simulink model "elevator"  (R2020a)
settings: Solver=VariableStepAuto  StartTime=0.0  StopTime=inf  RelTol=1e-3
PreLoadFcn:
  | slplc.api.loadDataTypes;
undefined symbols (not defined in the file): BOOL, DINT, INT, slplc
libraries: simulink x1
(part 1 of 38)
settings Model: Creator=Ishmael  LastModifiedBy=ieatg

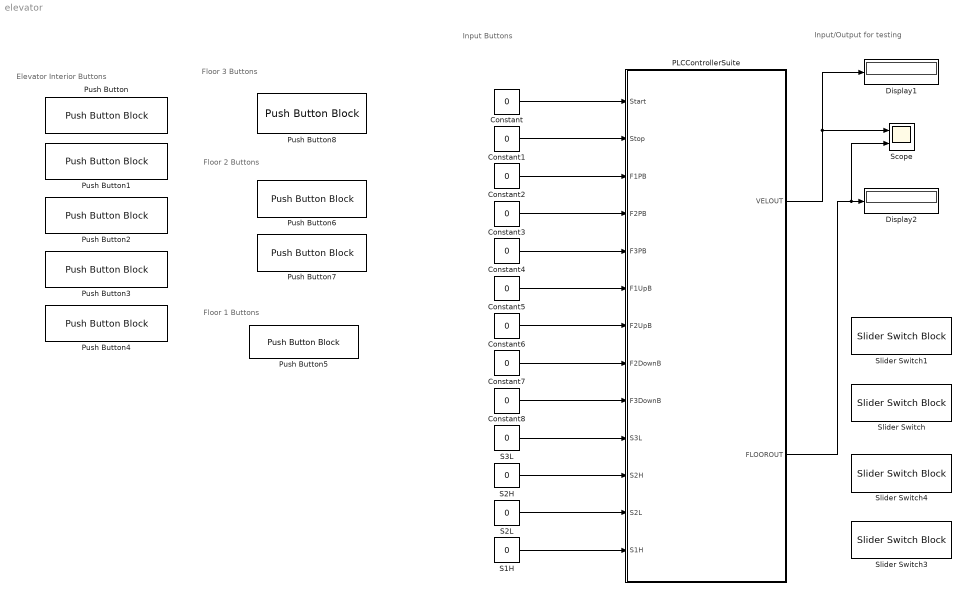
== system elevator ==
  note: Input/Output for testing
  note: Input Buttons
  note: Floor 2 Buttons
  note: Floor 3 Buttons
  note: Floor 1 Buttons
  note: Elevator Interior Buttons
  Constant{,1..8} (9 alike) : Constant  Value=0  OutDataTypeStr=BOOL
  Display1 : Display
  Display2 : Display
  PLCControllerSuite : Subsystem  TreatAsAtomicUnit=on  mask{PLCBlockType=PLCController, PLCPOUType=PLC Controller}
      mask init:
      | slplc.callbacks.initController(gcb);
      settings: OpenFcn=slplc.callbacks.openPOUBlock(gcb);
      mask Help: web([docroot '/plccoder/ref/plccontrollersuite' '.html']);
      mask DialogControl PLCBlockTitle Prompt: PLC Controller Block
  Push Button : PushButtonBlock  ButtonText=StartButton
  Push Button1 : PushButtonBlock  ButtonText=Stop
  Push Button2 : PushButtonBlock  ButtonText=Floor 1 PB
  Push Button3 : PushButtonBlock  ButtonText=Floor 2 PB
  Push Button4 : PushButtonBlock  ButtonText=Floor 3 PB
  Push Button5 : PushButtonBlock  ButtonText=Up Button Floor 1
  Push Button6 : PushButtonBlock  ButtonText=Up Button Floor 2
  Push Button7 : PushButtonBlock  ButtonText=Down Button Floor 2
  Push Button8 : PushButtonBlock  ButtonText=Down Button Floor 3
  S1H : Constant  Value=0  OutDataTypeStr=BOOL
  S2H : Constant  Value=0  OutDataTypeStr=BOOL
  S2L : Constant  Value=0  OutDataTypeStr=BOOL
  S3L : Constant  Value=0  OutDataTypeStr=BOOL
  Scope : Scope  NumInputPorts=2
  Slider Switch{,1,3..4} (4 alike) : SliderSwitchBlock
      settings: Values={{'Off', 'On'}, [0 1]}
  wires:
  Constant/1 -> PLCControllerSuite/1(Start)
  Constant1/1 -> PLCControllerSuite/2(Stop)
  Constant2/1 -> PLCControllerSuite/3(F1PB)
  Constant3/1 -> PLCControllerSuite/4(F2PB)
  Constant4/1 -> PLCControllerSuite/5(F3PB)
  Constant5/1 -> PLCControllerSuite/6(F1UpB)
  Constant6/1 -> PLCControllerSuite/7(F2UpB)
  Constant8/1 -> PLCControllerSuite/9(F3DownB)
  Constant7/1 -> PLCControllerSuite/8(F2DownB)
  PLCControllerSuite/1(VELOUT) -> Display1/1, Scope/1
  S3L/1 -> PLCControllerSuite/10(S3L)
  S2H/1 -> PLCControllerSuite/11(S2H)
  S2L/1 -> PLCControllerSuite/12(S2L)
  S1H/1 -> PLCControllerSuite/13(S1H)
  PLCControllerSuite/2(FLOOROUT) -> Scope/2, Display2/1

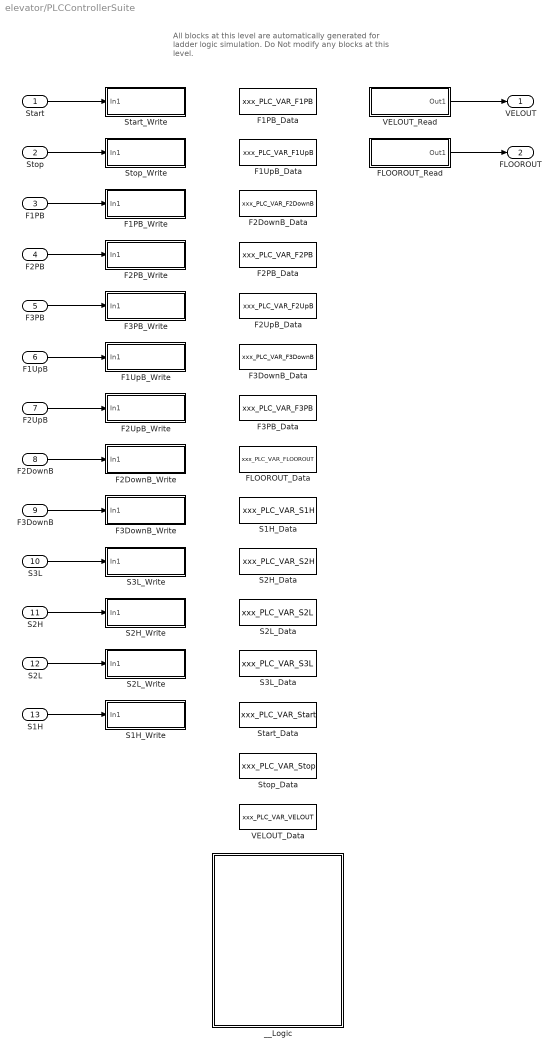
== system elevator/PLCControllerSuite ==
  note: All blocks at this level are automatically generated for ladder logic simulation.
      | Do Not modify any blocks at this level.
  Start : Inport  OutDataTypeStr=BOOL
  Stop : Inport  Port=2  OutDataTypeStr=BOOL
  F1PB : Inport  Port=3  OutDataTypeStr=BOOL
  F2PB : Inport  Port=4  OutDataTypeStr=BOOL
  F3PB : Inport  Port=5  OutDataTypeStr=BOOL
  F1UpB : Inport  Port=6  OutDataTypeStr=BOOL
  F2UpB : Inport  Port=7  OutDataTypeStr=BOOL
  F2DownB : Inport  Port=8  OutDataTypeStr=BOOL
  F3DownB : Inport  Port=9  OutDataTypeStr=BOOL
  S3L : Inport  Port=10  OutDataTypeStr=BOOL
  S2H : Inport  Port=11  OutDataTypeStr=BOOL
  S2L : Inport  Port=12  OutDataTypeStr=BOOL
  S1H : Inport  Port=13  OutDataTypeStr=BOOL
  F1PB_Data : DataStoreMemory  Tag=POUVariable  Priority=10  DataStoreName=xxx_PLC_VAR_F1PB  ShowAdditionalParam=off  OutDataTypeStr=BOOL  Dimensions=1
  F1PB_Write : Subsystem  Priority=11  DisableCoverage=on  TreatAsAtomicUnit=on  mask{PLCOperandTag=F1PB, PLCOperandExpression=xxx_PLC_VAR_F1PB, PLCBlockType=VarWrite, PLCPOUType=VarWrite}
      mask prompts: PLCOperandTag "Operand Tag:"
      mask init:
      | slplc.callbacks.initInstruction(gcb);
      mask Help: web([docroot '/plccoder/ref/varwrite' '.html']);
      mask DialogControl PLCBlockTitle Prompt: Variable Write
      mask Display: disp(get_param(gcb, 'PLCOperandTag'));
  F1UpB_Data : DataStoreMemory  Tag=POUVariable  Priority=10  DataStoreName=xxx_PLC_VAR_F1UpB  ShowAdditionalParam=off  OutDataTypeStr=BOOL  Dimensions=1
  F1UpB_Write : Subsystem  Priority=11  DisableCoverage=on  TreatAsAtomicUnit=on  mask{PLCOperandTag=F1UpB, PLCOperandExpression=xxx_PLC_VAR_F1UpB, PLCBlockType=VarWrite, PLCPOUType=VarWrite}
      mask prompts: PLCOperandTag "Operand Tag:"
      mask init:
      | slplc.callbacks.initInstruction(gcb);
      mask Help: web([docroot '/plccoder/ref/varwrite' '.html']);
      mask DialogControl PLCBlockTitle Prompt: Variable Write
      mask Display: disp(get_param(gcb, 'PLCOperandTag'));
  F2DownB_Data : DataStoreMemory  Tag=POUVariable  Priority=10  DataStoreName=xxx_PLC_VAR_F2DownB  ShowAdditionalParam=off  OutDataTypeStr=BOOL  Dimensions=1
  F2DownB_Write : Subsystem  Priority=11  DisableCoverage=on  TreatAsAtomicUnit=on  mask{PLCOperandTag=F2DownB, PLCOperandExpression=xxx_PLC_VAR_F2DownB, PLCBlockType=VarWrite, PLCPOUType=VarWrite}
      mask prompts: PLCOperandTag "Operand Tag:"
      mask init:
      | slplc.callbacks.initInstruction(gcb);
      mask Help: web([docroot '/plccoder/ref/varwrite' '.html']);
      mask DialogControl PLCBlockTitle Prompt: Variable Write
      mask Display: disp(get_param(gcb, 'PLCOperandTag'));
  F2PB_Data : DataStoreMemory  Tag=POUVariable  Priority=10  DataStoreName=xxx_PLC_VAR_F2PB  ShowAdditionalParam=off  OutDataTypeStr=BOOL  Dimensions=1
  F2PB_Write : Subsystem  Priority=11  DisableCoverage=on  TreatAsAtomicUnit=on  mask{PLCOperandTag=F2PB, PLCOperandExpression=xxx_PLC_VAR_F2PB, PLCBlockType=VarWrite, PLCPOUType=VarWrite}
      mask prompts: PLCOperandTag "Operand Tag:"
      mask init:
      | slplc.callbacks.initInstruction(gcb);
      mask Help: web([docroot '/plccoder/ref/varwrite' '.html']);
      mask DialogControl PLCBlockTitle Prompt: Variable Write
      mask Display: disp(get_param(gcb, 'PLCOperandTag'));
  F2UpB_Data : DataStoreMemory  Tag=POUVariable  Priority=10  DataStoreName=xxx_PLC_VAR_F2UpB  ShowAdditionalParam=off  OutDataTypeStr=BOOL  Dimensions=1
  F2UpB_Write : Subsystem  Priority=11  DisableCoverage=on  TreatAsAtomicUnit=on  mask{PLCOperandTag=F2UpB, PLCOperandExpression=xxx_PLC_VAR_F2UpB, PLCBlockType=VarWrite, PLCPOUType=VarWrite}
      mask prompts: PLCOperandTag "Operand Tag:"
      mask init:
      | slplc.callbacks.initInstruction(gcb);
      mask Help: web([docroot '/plccoder/ref/varwrite' '.html']);
      mask DialogControl PLCBlockTitle Prompt: Variable Write
      mask Display: disp(get_param(gcb, 'PLCOperandTag'));
  F3DownB_Data : DataStoreMemory  Tag=POUVariable  Priority=10  DataStoreName=xxx_PLC_VAR_F3DownB  ShowAdditionalParam=off  OutDataTypeStr=BOOL  Dimensions=1
  F3DownB_Write : Subsystem  Priority=11  DisableCoverage=on  TreatAsAtomicUnit=on  mask{PLCOperandTag=F3DownB, PLCOperandExpression=xxx_PLC_VAR_F3DownB, PLCBlockType=VarWrite, PLCPOUType=VarWrite}
      mask prompts: PLCOperandTag "Operand Tag:"
      mask init:
      | slplc.callbacks.initInstruction(gcb);
      mask Help: web([docroot '/plccoder/ref/varwrite' '.html']);
      mask DialogControl PLCBlockTitle Prompt: Variable Write
      mask Display: disp(get_param(gcb, 'PLCOperandTag'));
  F3PB_Data : DataStoreMemory  Tag=POUVariable  Priority=10  DataStoreName=xxx_PLC_VAR_F3PB  ShowAdditionalParam=off  OutDataTypeStr=BOOL  Dimensions=1
  F3PB_Write : Subsystem  Priority=11  DisableCoverage=on  TreatAsAtomicUnit=on  mask{PLCOperandTag=F3PB, PLCOperandExpression=xxx_PLC_VAR_F3PB, PLCBlockType=VarWrite, PLCPOUType=VarWrite}
      mask prompts: PLCOperandTag "Operand Tag:"
      mask init:
      | slplc.callbacks.initInstruction(gcb);
      mask Help: web([docroot '/plccoder/ref/varwrite' '.html']);
      mask DialogControl PLCBlockTitle Prompt: Variable Write
      mask Display: disp(get_param(gcb, 'PLCOperandTag'));
  FLOOROUT_Data : DataStoreMemory  Tag=POUVariable  Priority=10  DataStoreName=xxx_PLC_VAR_FLOOROUT  ShowAdditionalParam=off  OutDataTypeStr=INT  Dimensions=1
  FLOOROUT_Read : Subsystem  Priority=13  DisableCoverage=on  TreatAsAtomicUnit=on  mask{PLCOperandTag=FLOOROUT, PLCOperandExpression=xxx_PLC_VAR_FLOOROUT, PLCBlockType=VarRead, PLCPOUType=VarRead}
      mask prompts: PLCOperandTag "Operand Tag"
      mask init:
      | block = gcb;
      | maskObj = Simulink.Mask.get(block);
      | maskObj.Display = sprintf('disp(''%s'');', PLCOperandTag);
      | slplc.callbacks.initInstruction(gcb);
      mask Help: web([docroot '/plccoder/ref/varread' '.html']);
      mask DialogControl PLCBlockTitle Prompt: Variable Read
      mask Display: disp('FLOOROUT');
  S1H_Data : DataStoreMemory  Tag=POUVariable  Priority=10  DataStoreName=xxx_PLC_VAR_S1H  ShowAdditionalParam=off  OutDataTypeStr=BOOL  Dimensions=1
  S1H_Write : Subsystem  Priority=11  DisableCoverage=on  TreatAsAtomicUnit=on  mask{PLCOperandTag=S1H, PLCOperandExpression=xxx_PLC_VAR_S1H, PLCBlockType=VarWrite, PLCPOUType=VarWrite}
      mask prompts: PLCOperandTag "Operand Tag:"
      mask init:
      | slplc.callbacks.initInstruction(gcb);
      mask Help: web([docroot '/plccoder/ref/varwrite' '.html']);
      mask DialogControl PLCBlockTitle Prompt: Variable Write
      mask Display: disp(get_param(gcb, 'PLCOperandTag'));
  S2H_Data : DataStoreMemory  Tag=POUVariable  Priority=10  DataStoreName=xxx_PLC_VAR_S2H  ShowAdditionalParam=off  OutDataTypeStr=BOOL  Dimensions=1
  S2H_Write : Subsystem  Priority=11  DisableCoverage=on  TreatAsAtomicUnit=on  mask{PLCOperandTag=S2H, PLCOperandExpression=xxx_PLC_VAR_S2H, PLCBlockType=VarWrite, PLCPOUType=VarWrite}
      mask prompts: PLCOperandTag "Operand Tag:"
      mask init:
      | slplc.callbacks.initInstruction(gcb);
      mask Help: web([docroot '/plccoder/ref/varwrite' '.html']);
      mask DialogControl PLCBlockTitle Prompt: Variable Write
      mask Display: disp(get_param(gcb, 'PLCOperandTag'));
  S2L_Data : DataStoreMemory  Tag=POUVariable  Priority=10  DataStoreName=xxx_PLC_VAR_S2L  ShowAdditionalParam=off  OutDataTypeStr=BOOL  Dimensions=1
  S2L_Write : Subsystem  Priority=11  DisableCoverage=on  TreatAsAtomicUnit=on  mask{PLCOperandTag=S2L, PLCOperandExpression=xxx_PLC_VAR_S2L, PLCBlockType=VarWrite, PLCPOUType=VarWrite}
      mask prompts: PLCOperandTag "Operand Tag:"
      mask init:
      | slplc.callbacks.initInstruction(gcb);
      mask Help: web([docroot '/plccoder/ref/varwrite' '.html']);
      mask DialogControl PLCBlockTitle Prompt: Variable Write
      mask Display: disp(get_param(gcb, 'PLCOperandTag'));
  S3L_Data : DataStoreMemory  Tag=POUVariable  Priority=10  DataStoreName=xxx_PLC_VAR_S3L  ShowAdditionalParam=off  OutDataTypeStr=BOOL  Dimensions=1
  S3L_Write : Subsystem  Priority=11  DisableCoverage=on  TreatAsAtomicUnit=on  mask{PLCOperandTag=S3L, PLCOperandExpression=xxx_PLC_VAR_S3L, PLCBlockType=VarWrite, PLCPOUType=VarWrite}
      mask prompts: PLCOperandTag "Operand Tag:"
      mask init:
      | slplc.callbacks.initInstruction(gcb);
      mask Help: web([docroot '/plccoder/ref/varwrite' '.html']);
      mask DialogControl PLCBlockTitle Prompt: Variable Write
      mask Display: disp(get_param(gcb, 'PLCOperandTag'));
  Start_Data : DataStoreMemory  Tag=POUVariable  Priority=10  DataStoreName=xxx_PLC_VAR_Start  ShowAdditionalParam=off  OutDataTypeStr=BOOL  Dimensions=1
  Start_Write : Subsystem  Priority=11  DisableCoverage=on  TreatAsAtomicUnit=on  mask{PLCOperandTag=Start, PLCOperandExpression=xxx_PLC_VAR_Start, PLCBlockType=VarWrite, PLCPOUType=VarWrite}
      mask prompts: PLCOperandTag "Operand Tag:"
      mask init:
      | slplc.callbacks.initInstruction(gcb);
      mask Help: web([docroot '/plccoder/ref/varwrite' '.html']);
      mask DialogControl PLCBlockTitle Prompt: Variable Write
      mask Display: disp(get_param(gcb, 'PLCOperandTag'));
  Stop_Data : DataStoreMemory  Tag=POUVariable  Priority=10  DataStoreName=xxx_PLC_VAR_Stop  ShowAdditionalParam=off  OutDataTypeStr=BOOL  Dimensions=1
  Stop_Write : Subsystem  Priority=11  DisableCoverage=on  TreatAsAtomicUnit=on  mask{PLCOperandTag=Stop, PLCOperandExpression=xxx_PLC_VAR_Stop, PLCBlockType=VarWrite, PLCPOUType=VarWrite}
      mask prompts: PLCOperandTag "Operand Tag:"
      mask init:
      | slplc.callbacks.initInstruction(gcb);
      mask Help: web([docroot '/plccoder/ref/varwrite' '.html']);
      mask DialogControl PLCBlockTitle Prompt: Variable Write
      mask Display: disp(get_param(gcb, 'PLCOperandTag'));
  VELOUT_Data : DataStoreMemory  Tag=POUVariable  Priority=10  DataStoreName=xxx_PLC_VAR_VELOUT  InitialValue=0.0  ShowAdditionalParam=off  OutDataTypeStr=single  Dimensions=1
  VELOUT_Read : Subsystem  Priority=13  DisableCoverage=on  TreatAsAtomicUnit=on  mask{PLCOperandTag=VELOUT, PLCOperandExpression=xxx_PLC_VAR_VELOUT, PLCBlockType=VarRead, PLCPOUType=VarRead}
      mask prompts: PLCOperandTag "Operand Tag"
      mask init:
      | block = gcb;
      | maskObj = Simulink.Mask.get(block);
      | maskObj.Display = sprintf('disp(''%s'');', PLCOperandTag);
      | slplc.callbacks.initInstruction(gcb);
      mask Help: web([docroot '/plccoder/ref/varread' '.html']);
      mask DialogControl PLCBlockTitle Prompt: Variable Read
      mask Display: disp('VELOUT');
  __Logic : Subsystem  Priority=12  TreatAsAtomicUnit=on
  VELOUT : Outport
  FLOOROUT : Outport  Port=2
  wires:
  Start/1 -> Start_Write/1(In1)
  Stop/1 -> Stop_Write/1(In1)
  F1PB/1 -> F1PB_Write/1(In1)
  F2PB/1 -> F2PB_Write/1(In1)
  F3PB/1 -> F3PB_Write/1(In1)
  F1UpB/1 -> F1UpB_Write/1(In1)
  F2DownB/1 -> F2DownB_Write/1(In1)
  F2UpB/1 -> F2UpB_Write/1(In1)
  F3DownB/1 -> F3DownB_Write/1(In1)
  S1H/1 -> S1H_Write/1(In1)
  S2H/1 -> S2H_Write/1(In1)
  S2L/1 -> S2L_Write/1(In1)
  S3L/1 -> S3L_Write/1(In1)
  VELOUT_Read/1(Out1) -> VELOUT/1
  FLOOROUT_Read/1(Out1) -> FLOOROUT/1

== system elevator/PLCControllerSuite/F1PB_Write ==
  In1 : Inport
  __CoreVarWrite : Subsystem  Tag=CoreVarWriteBlock  DisableCoverage=on  TreatAsAtomicUnit=on  mask{PLCBlockType=CoreVarWrite}
      mask init:
      | slplc.callbacks.initCoreVariable(gcb, 'write');
      mask DialogControl PLCBlockTitle Prompt: Core Variable Write
  wires:
  In1/1 -> __CoreVarWrite/1(u)

== system elevator/PLCControllerSuite/F1UpB_Write ==
  In1 : Inport
  __CoreVarWrite : Subsystem  Tag=CoreVarWriteBlock  DisableCoverage=on  TreatAsAtomicUnit=on  mask{PLCBlockType=CoreVarWrite}
      mask init:
      | slplc.callbacks.initCoreVariable(gcb, 'write');
      mask DialogControl PLCBlockTitle Prompt: Core Variable Write
  wires:
  In1/1 -> __CoreVarWrite/1(u)

== system elevator/PLCControllerSuite/F2DownB_Write ==
  In1 : Inport
  __CoreVarWrite : Subsystem  Tag=CoreVarWriteBlock  DisableCoverage=on  TreatAsAtomicUnit=on  mask{PLCBlockType=CoreVarWrite}
      mask init:
      | slplc.callbacks.initCoreVariable(gcb, 'write');
      mask DialogControl PLCBlockTitle Prompt: Core Variable Write
  wires:
  In1/1 -> __CoreVarWrite/1(u)

== system elevator/PLCControllerSuite/F2PB_Write ==
  In1 : Inport
  __CoreVarWrite : Subsystem  Tag=CoreVarWriteBlock  DisableCoverage=on  TreatAsAtomicUnit=on  mask{PLCBlockType=CoreVarWrite}
      mask init:
      | slplc.callbacks.initCoreVariable(gcb, 'write');
      mask DialogControl PLCBlockTitle Prompt: Core Variable Write
  wires:
  In1/1 -> __CoreVarWrite/1(u)

== system elevator/PLCControllerSuite/F2UpB_Write ==
  In1 : Inport
  __CoreVarWrite : Subsystem  Tag=CoreVarWriteBlock  DisableCoverage=on  TreatAsAtomicUnit=on  mask{PLCBlockType=CoreVarWrite}
      mask init:
      | slplc.callbacks.initCoreVariable(gcb, 'write');
      mask DialogControl PLCBlockTitle Prompt: Core Variable Write
  wires:
  In1/1 -> __CoreVarWrite/1(u)

== system elevator/PLCControllerSuite/F3DownB_Write ==
  In1 : Inport
  __CoreVarWrite : Subsystem  Tag=CoreVarWriteBlock  DisableCoverage=on  TreatAsAtomicUnit=on  mask{PLCBlockType=CoreVarWrite}
      mask init:
      | slplc.callbacks.initCoreVariable(gcb, 'write');
      mask DialogControl PLCBlockTitle Prompt: Core Variable Write
  wires:
  In1/1 -> __CoreVarWrite/1(u)

== system elevator/PLCControllerSuite/F3PB_Write ==
  In1 : Inport
  __CoreVarWrite : Subsystem  Tag=CoreVarWriteBlock  DisableCoverage=on  TreatAsAtomicUnit=on  mask{PLCBlockType=CoreVarWrite}
      mask init:
      | slplc.callbacks.initCoreVariable(gcb, 'write');
      mask DialogControl PLCBlockTitle Prompt: Core Variable Write
  wires:
  In1/1 -> __CoreVarWrite/1(u)

== system elevator/PLCControllerSuite/FLOOROUT_Read ==
  __CoreVarRead : Subsystem  Tag=CoreVarReadBlock  DisableCoverage=on  TreatAsAtomicUnit=on  mask{PLCBlockType=CoreVarRead}
      mask init:
      | slplc.callbacks.initCoreVariable(gcb, 'read');
      mask DialogControl PLCBlockTitle Prompt: Core Variable Read
  Out1 : Outport  VectorParamsAs1DForOutWhenUnconnected=off
  wires:
  __CoreVarRead/1(y) -> Out1/1

== system elevator/PLCControllerSuite/S1H_Write ==
  In1 : Inport
  __CoreVarWrite : Subsystem  Tag=CoreVarWriteBlock  DisableCoverage=on  TreatAsAtomicUnit=on  mask{PLCBlockType=CoreVarWrite}
      mask init:
      | slplc.callbacks.initCoreVariable(gcb, 'write');
      mask DialogControl PLCBlockTitle Prompt: Core Variable Write
  wires:
  In1/1 -> __CoreVarWrite/1(u)

== system elevator/PLCControllerSuite/S2H_Write ==
  In1 : Inport
  __CoreVarWrite : Subsystem  Tag=CoreVarWriteBlock  DisableCoverage=on  TreatAsAtomicUnit=on  mask{PLCBlockType=CoreVarWrite}
      mask init:
      | slplc.callbacks.initCoreVariable(gcb, 'write');
      mask DialogControl PLCBlockTitle Prompt: Core Variable Write
  wires:
  In1/1 -> __CoreVarWrite/1(u)

== system elevator/PLCControllerSuite/S2L_Write ==
  In1 : Inport
  __CoreVarWrite : Subsystem  Tag=CoreVarWriteBlock  DisableCoverage=on  TreatAsAtomicUnit=on  mask{PLCBlockType=CoreVarWrite}
      mask init:
      | slplc.callbacks.initCoreVariable(gcb, 'write');
      mask DialogControl PLCBlockTitle Prompt: Core Variable Write
  wires:
  In1/1 -> __CoreVarWrite/1(u)

== system elevator/PLCControllerSuite/S3L_Write ==
  In1 : Inport
  __CoreVarWrite : Subsystem  Tag=CoreVarWriteBlock  DisableCoverage=on  TreatAsAtomicUnit=on  mask{PLCBlockType=CoreVarWrite}
      mask init:
      | slplc.callbacks.initCoreVariable(gcb, 'write');
      mask DialogControl PLCBlockTitle Prompt: Core Variable Write
  wires:
  In1/1 -> __CoreVarWrite/1(u)

== system elevator/PLCControllerSuite/Start_Write ==
  In1 : Inport
  __CoreVarWrite : Subsystem  Tag=CoreVarWriteBlock  DisableCoverage=on  TreatAsAtomicUnit=on  mask{PLCBlockType=CoreVarWrite}
      mask init:
      | slplc.callbacks.initCoreVariable(gcb, 'write');
      mask DialogControl PLCBlockTitle Prompt: Core Variable Write
  wires:
  In1/1 -> __CoreVarWrite/1(u)

== system elevator/PLCControllerSuite/Stop_Write ==
  In1 : Inport
  __CoreVarWrite : Subsystem  Tag=CoreVarWriteBlock  DisableCoverage=on  TreatAsAtomicUnit=on  mask{PLCBlockType=CoreVarWrite}
      mask init:
      | slplc.callbacks.initCoreVariable(gcb, 'write');
      mask DialogControl PLCBlockTitle Prompt: Core Variable Write
  wires:
  In1/1 -> __CoreVarWrite/1(u)

== system elevator/PLCControllerSuite/VELOUT_Read ==
  __CoreVarRead : Subsystem  Tag=CoreVarReadBlock  DisableCoverage=on  TreatAsAtomicUnit=on  mask{PLCBlockType=CoreVarRead}
      mask init:
      | slplc.callbacks.initCoreVariable(gcb, 'read');
      mask DialogControl PLCBlockTitle Prompt: Core Variable Read
  Out1 : Outport  VectorParamsAs1DForOutWhenUnconnected=off
  wires:
  __CoreVarRead/1(y) -> Out1/1

== system elevator/PLCControllerSuite/__Logic ==
  Controller Tags : Subsystem  Tag=ControllerVariableSS  DisableCoverage=on  TreatAsAtomicUnit=on  mask{PLCVarStartName=Start, PLCVarStartAddress=<empty>, PLCVarStartMapping=Input Symbol, PLCVarStartPortIndex=1, PLCVarStartDataType=BOOL, PLCVarStartSize=1, PLCVarStartInitialValue=0, PLCVarStartToDelete=off, PLCVarStopName=Stop, PLCVarStopAddress=<empty>, PLCVarStopMapping=Input Symbol, PLCVarStopPortIndex=2, PLCVarStopDataType=BOOL, PLCVarStopSize=1, PLCVarStopInitialValue=0, PLCVarStopToDelete=off, PLCVarF1PBName=F1PB, PLCVarF1PBAddress=<empty>, PLCVarF1PBMapping=Input Symbol, PLCVarF1PBPortIndex=3, PLCVarF1PBDataType=BOOL, PLCVarF1PBSize=1, PLCVarF1PBInitialValue=0, PLCVarF1PBToDelete=off, PLCVarF2PBName=F2PB, PLCVarF2PBAddress=<empty>, PLCVarF2PBMapping=Input Symbol, PLCVarF2PBPortIndex=4, PLCVarF2PBDataType=BOOL, PLCVarF2PBSize=1, PLCVarF2PBInitialValue=0, PLCVarF2PBToDelete=off, PLCVarF3PBName=F3PB, PLCVarF3PBAddress=<empty>, PLCVarF3PBMapping=Input Symbol, PLCVarF3PBPortIndex=5, PLCVarF3PBDataType=BOOL, PLCVarF3PBSize=1, PLCVarF3PBInitialValue=0, PLCVarF3PBToDelete=off, PLCVarF1UpBName=F1UpB, PLCVarF1UpBAddress=<empty>, PLCVarF1UpBMapping=Input Symbol, PLCVarF1UpBPortIndex=6, PLCVarF1UpBDataType=BOOL, PLCVarF1UpBSize=1, PLCVarF1UpBInitialValue=0, PLCVarF1UpBToDelete=off, PLCVarF2UpBName=F2UpB, PLCVarF2UpBAddress=<empty>, PLCVarF2UpBMapping=Input Symbol, PLCVarF2UpBPortIndex=7, PLCVarF2UpBDataType=BOOL, PLCVarF2UpBSize=1, PLCVarF2UpBInitialValue=0, PLCVarF2UpBToDelete=off, PLCVarF2DownBName=F2DownB, PLCVarF2DownBAddress=<empty>, PLCVarF2DownBMapping=Input Symbol, PLCVarF2DownBPortIndex=8, PLCVarF2DownBDataType=BOOL, PLCVarF2DownBSize=1, PLCVarF2DownBInitialValue=0, PLCVarF2DownBToDelete=off, PLCVarF3DownBName=F3DownB, PLCVarF3DownBAddress=<empty>, PLCVarF3DownBMapping=Input Symbol, PLCVarF3DownBPortIndex=9, PLCVarF3DownBDataType=BOOL, PLCVarF3DownBSize=1, PLCVarF3DownBInitialValue=0, PLCVarF3DownBToDelete=off, PLCVarS3LName=S3L, PLCVarS3LAddress=<empty>, PLCVarS3LMapping=Input Symbol, PLCVarS3LPortIndex=10, PLCVarS3LDataType=BOOL, PLCVarS3LSize=1, PLCVarS3LInitialValue=0, PLCVarS3LToDelete=off, PLCVarS2HName=S2H, PLCVarS2HAddress=<empty>, PLCVarS2HMapping=Input Symbol, PLCVarS2HPortIndex=11, PLCVarS2HDataType=BOOL, PLCVarS2HSize=1, PLCVarS2HInitialValue=0, PLCVarS2HToDelete=off, PLCVarS2LName=S2L, PLCVarS2LAddress=<empty>, PLCVarS2LMapping=Input Symbol, PLCVarS2LPortIndex=12, PLCVarS2LDataType=BOOL, PLCVarS2LSize=1, PLCVarS2LInitialValue=0, PLCVarS2LToDelete=off, PLCVarS1HName=S1H, PLCVarS1HAddress=<empty>, PLCVarS1HMapping=Input Symbol, PLCVarS1HPortIndex=13, PLCVarS1HDataType=BOOL, PLCVarS1HSize=1, PLCVarS1HInitialValue=0, PLCVarS1HToDelete=off, PLCVarVELOUTName=VELOUT, PLCVarVELOUTAddress=<empty>, PLCVarVELOUTMapping=Output Symbol, PLCVarVELOUTPortIndex=1, PLCVarVELOUTDataType=single, PLCVarVELOUTSize=1, PLCVarVELOUTInitialValue=0.0, PLCVarVELOUTToDelete=off, PLCVarFLOOROUTName=FLOOROUT, PLCVarFLOOROUTAddress=<empty>, PLCVarFLOOROUTMapping=Output Symbol, PLCVarFLOOROUTPortIndex=2, PLCVarFLOOROUTDataType=INT, PLCVarFLOOROUTSize=1, PLCVarFLOOROUTInitialValue=0, PLCVarFLOOROUTToDelete=off}
      mask init:
      | slplc.callbacks.initControllerVarSS(gcb);
      settings: OpenFcn=slplc.callbacks.openControllerVariableSS(gcb);
      mask Help: web([docroot '/plccoder/ref/controllertags' '.html']);
      mask TypeOptions PLCVarStartMapping: Global Variable | Input Symbol | Output Symbol
      mask Callback PLCVarStartMapping: slplc.callbacks.updateControllerVarSS(gcb);
      mask TypeOptions PLCVarStartPortIndex: 1 | 2 | 3 | 4 | 5 | 6 | 7 | 8 | 9 | 10 | 11 | 12 | 13 | 14 | 15
      mask TypeOptions PLCVarStopMapping: Global Variable | Input Symbol | Output Symbol
      mask Callback PLCVarStopMapping: slplc.callbacks.updateControllerVarSS(gcb);
      mask TypeOptions PLCVarStopPortIndex: 1 | 2 | 3 | 4 | 5 | 6 | 7 | 8 | 9 | 10 | 11 | 12 | 13 | 14 | 15
      mask TypeOptions PLCVarF1PBMapping: Global Variable | Input Symbol | Output Symbol
      mask Callback PLCVarF1PBMapping: slplc.callbacks.updateControllerVarSS(gcb);
      mask TypeOptions PLCVarF1PBPortIndex: 1 | 2 | 3 | 4 | 5 | 6 | 7 | 8 | 9 | 10 | 11 | 12 | 13 | 14 | 15
      mask TypeOptions PLCVarF2PBMapping: Global Variable | Input Symbol | Output Symbol
      mask Callback PLCVarF2PBMapping: slplc.callbacks.updateControllerVarSS(gcb);
      mask TypeOptions PLCVarF2PBPortIndex: 1 | 2 | 3 | 4 | 5 | 6 | 7 | 8 | 9 | 10 | 11 | 12 | 13 | 14 | 15
      mask TypeOptions PLCVarF3PBMapping: Global Variable | Input Symbol | Output Symbol
      mask Callback PLCVarF3PBMapping: slplc.callbacks.updateControllerVarSS(gcb);
      mask TypeOptions PLCVarF3PBPortIndex: 1 | 2 | 3 | 4 | 5 | 6 | 7 | 8 | 9 | 10 | 11 | 12 | 13 | 14 | 15
      mask TypeOptions PLCVarF1UpBMapping: Global Variable | Input Symbol | Output Symbol
      mask Callback PLCVarF1UpBMapping: slplc.callbacks.updateControllerVarSS(gcb);
      mask TypeOptions PLCVarF1UpBPortIndex: 1 | 2 | 3 | 4 | 5 | 6 | 7 | 8 | 9 | 10 | 11 | 12 | 13 | 14 | 15
      mask TypeOptions PLCVarF2UpBMapping: Global Variable | Input Symbol | Output Symbol
      mask Callback PLCVarF2UpBMapping: slplc.callbacks.updateControllerVarSS(gcb);
      mask TypeOptions PLCVarF2UpBPortIndex: 1 | 2 | 3 | 4 | 5 | 6 | 7 | 8 | 9 | 10 | 11 | 12 | 13 | 14 | 15
      mask TypeOptions PLCVarF2DownBMapping: Global Variable | Input Symbol | Output Symbol
      mask Callback PLCVarF2DownBMapping: slplc.callbacks.updateControllerVarSS(gcb);
      mask TypeOptions PLCVarF2DownBPortIndex: 1 | 2 | 3 | 4 | 5 | 6 | 7 | 8 | 9 | 10 | 11 | 12 | 13 | 14 | 15
      mask TypeOptions PLCVarF3DownBMapping: Global Variable | Input Symbol | Output Symbol
      mask Callback PLCVarF3DownBMapping: slplc.callbacks.updateControllerVarSS(gcb);
      mask TypeOptions PLCVarF3DownBPortIndex: 1 | 2 | 3 | 4 | 5 | 6 | 7 | 8 | 9 | 10 | 11 | 12 | 13 | 14 | 15
      mask TypeOptions PLCVarS3LMapping: Global Variable | Input Symbol | Output Symbol
      mask Callback PLCVarS3LMapping: slplc.callbacks.updateControllerVarSS(gcb);
      mask TypeOptions PLCVarS3LPortIndex: 1 | 2 | 3 | 4 | 5 | 6 | 7 | 8 | 9 | 10 | 11 | 12 | 13 | 14 | 15
      mask TypeOptions PLCVarS2HMapping: Global Variable | Input Symbol | Output Symbol
      mask Callback PLCVarS2HMapping: slplc.callbacks.updateControllerVarSS(gcb);
      mask TypeOptions PLCVarS2HPortIndex: 1 | 2 | 3 | 4 | 5 | 6 | 7 | 8 | 9 | 10 | 11 | 12 | 13 | 14 | 15
      mask TypeOptions PLCVarS2LMapping: Global Variable | Input Symbol | Output Symbol
      mask Callback PLCVarS2LMapping: slplc.callbacks.updateControllerVarSS(gcb);
      mask TypeOptions PLCVarS2LPortIndex: 1 | 2 | 3 | 4 | 5 | 6 | 7 | 8 | 9 | 10 | 11 | 12 | 13 | 14 | 15
      mask TypeOptions PLCVarS1HMapping: Global Variable | Input Symbol | Output Symbol
      mask Callback PLCVarS1HMapping: slplc.callbacks.updateControllerVarSS(gcb);
      mask TypeOptions PLCVarS1HPortIndex: 1 | 2 | 3 | 4 | 5 | 6 | 7 | 8 | 9 | 10 | 11 | 12 | 13 | 14 | 15
      mask TypeOptions PLCVarVELOUTMapping: Global Variable | Input Symbol | Output Symbol
      mask Callback PLCVarVELOUTMapping: slplc.callbacks.updateControllerVarSS(gcb);
      mask TypeOptions PLCVarVELOUTPortIndex: 1 | 2 | 3 | 4 | 5 | 6 | 7 | 8 | 9 | 10 | 11 | 12 | 13 | 14 | 15
      mask TypeOptions PLCVarFLOOROUTMapping: Global Variable | Input Symbol | Output Symbol
      mask Callback PLCVarFLOOROUTMapping: slplc.callbacks.updateControllerVarSS(gcb);
      mask TypeOptions PLCVarFLOOROUTPortIndex: 1 | 2 | 3 | 4 | 5 | 6 | 7 | 8 | 9 | 10 | 11 | 12 | 13 | 14 | 15
      mask DialogControl PLCBlockTitle Prompt: Global Variable and Symbol Spreadsheet
      mask DialogControl PLCVarListHeaderName Prompt: Name
      mask DialogControl PLCVarListHeaderAddress Prompt: Address (At)
      mask DialogControl PLCVarListHeaderMapping Prompt: Mapping Type
      mask DialogControl PLCVarListHeaderPortIndex Prompt: Port
      mask DialogControl PLCVarListHeaderDataType Prompt: Data Type
      mask DialogControl PLCVarListHeaderSize Prompt: Size
      mask DialogControl PLCVarListHeaderInitialValue Prompt: Initial Value
      mask DialogControl PLCVarListHeaderToDelete Prompt: Delete
  Task : Subsystem  TreatAsAtomicUnit=on  mask{PLCBlockType=Task, PLCPOUType=Task, PLCTaskWatchDog=0}
      settings: OpenFcn=slplc.callbacks.openTaskBlock(gcb);
      mask Help: web([docroot '/plccoder/ref/task' '.html']);
      mask DialogControl PLCBlockTitle Prompt: Task
  Up to Parent POU : Subsystem  DisableCoverage=on  TreatAsAtomicUnit=on  mask{PLCBlockType=OpenParentPOU}
      settings: OpenFcn=slplc.callbacks.openParentPOUBlock(gcb);
      mask Help: web([docroot '/plccoder/ref/uptoparentpou' '.html']);
      mask DialogControl PLCBlockTitle Prompt: Add Single Rung

== system elevator/PLCControllerSuite/F1PB_Write/__CoreVarWrite ==
  u : Inport
  DataWrite : DataStoreWrite  DataStoreName=xxx_PLC_VAR_F1PB
  wires:
  u/1 -> DataWrite/1

== system elevator/PLCControllerSuite/F1UpB_Write/__CoreVarWrite ==
  u : Inport
  DataWrite : DataStoreWrite  DataStoreName=xxx_PLC_VAR_F1UpB
  wires:
  u/1 -> DataWrite/1

== system elevator/PLCControllerSuite/F2DownB_Write/__CoreVarWrite ==
  u : Inport
  DataWrite : DataStoreWrite  DataStoreName=xxx_PLC_VAR_F2DownB
  wires:
  u/1 -> DataWrite/1

== system elevator/PLCControllerSuite/F2PB_Write/__CoreVarWrite ==
  u : Inport
  DataWrite : DataStoreWrite  DataStoreName=xxx_PLC_VAR_F2PB
  wires:
  u/1 -> DataWrite/1

== system elevator/PLCControllerSuite/F2UpB_Write/__CoreVarWrite ==
  u : Inport
  DataWrite : DataStoreWrite  DataStoreName=xxx_PLC_VAR_F2UpB
  wires:
  u/1 -> DataWrite/1

== system elevator/PLCControllerSuite/F3DownB_Write/__CoreVarWrite ==
  u : Inport
  DataWrite : DataStoreWrite  DataStoreName=xxx_PLC_VAR_F3DownB
  wires:
  u/1 -> DataWrite/1

== system elevator/PLCControllerSuite/F3PB_Write/__CoreVarWrite ==
  u : Inport
  DataWrite : DataStoreWrite  DataStoreName=xxx_PLC_VAR_F3PB
  wires:
  u/1 -> DataWrite/1

== system elevator/PLCControllerSuite/FLOOROUT_Read/__CoreVarRead ==
  DataRead : DataStoreRead  DataStoreName=xxx_PLC_VAR_FLOOROUT
  y : Outport  VectorParamsAs1DForOutWhenUnconnected=off
  wires:
  DataRead/1 -> y/1

== system elevator/PLCControllerSuite/S1H_Write/__CoreVarWrite ==
  u : Inport
  DataWrite : DataStoreWrite  DataStoreName=xxx_PLC_VAR_S1H
  wires:
  u/1 -> DataWrite/1

== system elevator/PLCControllerSuite/S2H_Write/__CoreVarWrite ==
  u : Inport
  DataWrite : DataStoreWrite  DataStoreName=xxx_PLC_VAR_S2H
  wires:
  u/1 -> DataWrite/1

== system elevator/PLCControllerSuite/S2L_Write/__CoreVarWrite ==
  u : Inport
  DataWrite : DataStoreWrite  DataStoreName=xxx_PLC_VAR_S2L
  wires:
  u/1 -> DataWrite/1

== system elevator/PLCControllerSuite/S3L_Write/__CoreVarWrite ==
  u : Inport
  DataWrite : DataStoreWrite  DataStoreName=xxx_PLC_VAR_S3L
  wires:
  u/1 -> DataWrite/1

== system elevator/PLCControllerSuite/Start_Write/__CoreVarWrite ==
  u : Inport
  DataWrite : DataStoreWrite  DataStoreName=xxx_PLC_VAR_Start
  wires:
  u/1 -> DataWrite/1

== system elevator/PLCControllerSuite/Stop_Write/__CoreVarWrite ==
  u : Inport
  DataWrite : DataStoreWrite  DataStoreName=xxx_PLC_VAR_Stop
  wires:
  u/1 -> DataWrite/1

== system elevator/PLCControllerSuite/VELOUT_Read/__CoreVarRead ==
  DataRead : DataStoreRead  DataStoreName=xxx_PLC_VAR_VELOUT
  y : Outport  VectorParamsAs1DForOutWhenUnconnected=off
  wires:
  DataRead/1 -> y/1

== system elevator/PLCControllerSuite/__Logic/Controller Tags ==

== system elevator/PLCControllerSuite/__Logic/Task ==
  Program : Subsystem  TreatAsAtomicUnit=on  mask{PLCPOUType=Program, PLCPOULanguage=LD, PLCBlockType=LDProgram}
      mask prompts: PLCPOUType "POU Type:"
      mask init:
      | slplc.callbacks.initProgram(gcb);
      settings: OpenFcn=slplc.callbacks.openPOUBlock(gcb);
      mask Help: web([docroot '/plccoder/ref/ldprogram' '.html']);
      mask DialogControl PLCBlockTitle Prompt: Program
      mask DialogControl PLCEditPOU Prompt: Edit POU
      mask DialogControl PLCEditInterface Prompt: Edit Variables
  Up to Parent POU : Subsystem  DisableCoverage=on  TreatAsAtomicUnit=on  mask{PLCBlockType=OpenParentPOU}
      settings: OpenFcn=slplc.callbacks.openParentPOUBlock(gcb);
      mask Help: web([docroot '/plccoder/ref/uptoparentpou' '.html']);
      mask DialogControl PLCBlockTitle Prompt: Add Single Rung

== system elevator/PLCControllerSuite/__Logic/Up to Parent POU ==

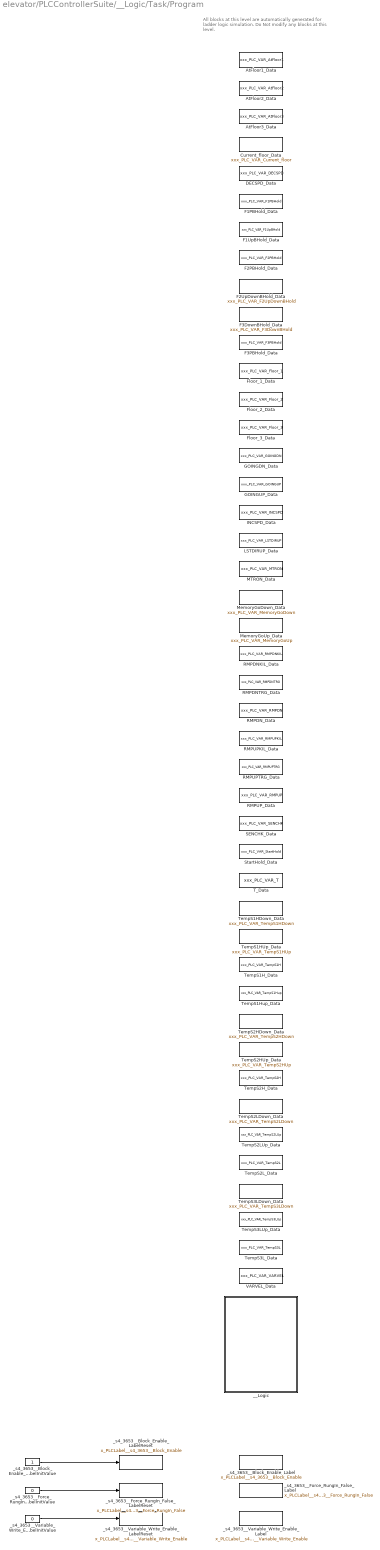
== system elevator/PLCControllerSuite/__Logic/Task/Program ==
  note: All blocks at this level are automatically generated for ladder logic simulation.
      | Do Not modify any blocks at this level.
  AtFloor1_Data : DataStoreMemory  Tag=POUVariable  Priority=10  DataStoreName=xxx_PLC_VAR_AtFloor1  InitialValue=false  ShowAdditionalParam=off  OutDataTypeStr=BOOL  Dimensions=1
  AtFloor2_Data : DataStoreMemory  Tag=POUVariable  Priority=10  DataStoreName=xxx_PLC_VAR_AtFloor2  InitialValue=false  ShowAdditionalParam=off  OutDataTypeStr=BOOL  Dimensions=1
  AtFloor3_Data : DataStoreMemory  Tag=POUVariable  Priority=10  DataStoreName=xxx_PLC_VAR_AtFloor3  InitialValue=false  ShowAdditionalParam=off  OutDataTypeStr=BOOL  Dimensions=1
  Current_floor_Data : DataStoreMemory  Tag=POUVariable  Priority=10  DataStoreName=xxx_PLC_VAR_Current_floor  InitialValue=1  ShowAdditionalParam=off  OutDataTypeStr=DINT  Dimensions=1
  DECSPD_Data : DataStoreMemory  Tag=POUVariable  Priority=10  DataStoreName=xxx_PLC_VAR_DECSPD  InitialValue=false  ShowAdditionalParam=off  OutDataTypeStr=BOOL  Dimensions=1
  F1PBHold_Data : DataStoreMemory  Tag=POUVariable  Priority=10  DataStoreName=xxx_PLC_VAR_F1PBHold  InitialValue=false  ShowAdditionalParam=off  OutDataTypeStr=BOOL  Dimensions=1
  F1UpBHold_Data : DataStoreMemory  Tag=POUVariable  Priority=10  DataStoreName=xxx_PLC_VAR_F1UpBHold  InitialValue=false  ShowAdditionalParam=off  OutDataTypeStr=BOOL  Dimensions=1
  F2PBHold_Data : DataStoreMemory  Tag=POUVariable  Priority=10  DataStoreName=xxx_PLC_VAR_F2PBHold  InitialValue=false  ShowAdditionalParam=off  OutDataTypeStr=BOOL  Dimensions=1
  F2UpDownBHold_Data : DataStoreMemory  Tag=POUVariable  Priority=10  DataStoreName=xxx_PLC_VAR_F2UpDownBHold  InitialValue=false  ShowAdditionalParam=off  OutDataTypeStr=BOOL  Dimensions=1
  F3DownBHold_Data : DataStoreMemory  Tag=POUVariable  Priority=10  DataStoreName=xxx_PLC_VAR_F3DownBHold  InitialValue=false  ShowAdditionalParam=off  OutDataTypeStr=BOOL  Dimensions=1
  F3PBHold_Data : DataStoreMemory  Tag=POUVariable  Priority=10  DataStoreName=xxx_PLC_VAR_F3PBHold  InitialValue=false  ShowAdditionalParam=off  OutDataTypeStr=BOOL  Dimensions=1
  Floor_1_Data : DataStoreMemory  Tag=POUVariable  Priority=10  DataStoreName=xxx_PLC_VAR_Floor_1  InitialValue=1  ShowAdditionalParam=off  OutDataTypeStr=DINT  Dimensions=1
  Floor_2_Data : DataStoreMemory  Tag=POUVariable  Priority=10  DataStoreName=xxx_PLC_VAR_Floor_2  InitialValue=2  ShowAdditionalParam=off  OutDataTypeStr=DINT  Dimensions=1
  Floor_3_Data : DataStoreMemory  Tag=POUVariable  Priority=10  DataStoreName=xxx_PLC_VAR_Floor_3  InitialValue=3  ShowAdditionalParam=off  OutDataTypeStr=DINT  Dimensions=1
  GOINGDN_Data : DataStoreMemory  Tag=POUVariable  Priority=10  DataStoreName=xxx_PLC_VAR_GOINGDN  InitialValue=false  ShowAdditionalParam=off  OutDataTypeStr=BOOL  Dimensions=1
  GOINGUP_Data : DataStoreMemory  Tag=POUVariable  Priority=10  DataStoreName=xxx_PLC_VAR_GOINGUP  InitialValue=false  ShowAdditionalParam=off  OutDataTypeStr=BOOL  Dimensions=1
  INCSPD_Data : DataStoreMemory  Tag=POUVariable  Priority=10  DataStoreName=xxx_PLC_VAR_INCSPD  InitialValue=false  ShowAdditionalParam=off  OutDataTypeStr=BOOL  Dimensions=1
  LSTDIRUP_Data : DataStoreMemory  Tag=POUVariable  Priority=10  DataStoreName=xxx_PLC_VAR_LSTDIRUP  InitialValue=false  ShowAdditionalParam=off  OutDataTypeStr=BOOL  Dimensions=1
  MTRON_Data : DataStoreMemory  Tag=POUVariable  Priority=10  DataStoreName=xxx_PLC_VAR_MTRON  InitialValue=false  ShowAdditionalParam=off  OutDataTypeStr=BOOL  Dimensions=1
  MemoryGoDown_Data : DataStoreMemory  Tag=POUVariable  Priority=10  DataStoreName=xxx_PLC_VAR_MemoryGoDown  InitialValue=false  ShowAdditionalParam=off  OutDataTypeStr=BOOL  Dimensions=1
  MemoryGoUp_Data : DataStoreMemory  Tag=POUVariable  Priority=10  DataStoreName=xxx_PLC_VAR_MemoryGoUp  InitialValue=false  ShowAdditionalParam=off  OutDataTypeStr=BOOL  Dimensions=1
  RMPDNKIL_Data : DataStoreMemory  Tag=POUVariable  Priority=10  DataStoreName=xxx_PLC_VAR_RMPDNKIL  InitialValue=false  ShowAdditionalParam=off  OutDataTypeStr=BOOL  Dimensions=1
  RMPDNTRG_Data : DataStoreMemory  Tag=POUVariable  Priority=10  DataStoreName=xxx_PLC_VAR_RMPDNTRG  InitialValue=false  ShowAdditionalParam=off  OutDataTypeStr=BOOL  Dimensions=1
  RMPDN_Data : DataStoreMemory  Tag=POUVariable  Priority=10  DataStoreName=xxx_PLC_VAR_RMPDN  InitialValue=false  ShowAdditionalParam=off  OutDataTypeStr=BOOL  Dimensions=1
  RMPUPKIL_Data : DataStoreMemory  Tag=POUVariable  Priority=10  DataStoreName=xxx_PLC_VAR_RMPUPKIL  InitialValue=false  ShowAdditionalParam=off  OutDataTypeStr=BOOL  Dimensions=1
  RMPUPTRG_Data : DataStoreMemory  Tag=POUVariable  Priority=10  DataStoreName=xxx_PLC_VAR_RMPUPTRG  InitialValue=false  ShowAdditionalParam=off  OutDataTypeStr=BOOL  Dimensions=1
  RMPUP_Data : DataStoreMemory  Tag=POUVariable  Priority=10  DataStoreName=xxx_PLC_VAR_RMPUP  InitialValue=false  ShowAdditionalParam=off  OutDataTypeStr=BOOL  Dimensions=1
  SENCHK_Data : DataStoreMemory  Tag=POUVariable  Priority=10  DataStoreName=xxx_PLC_VAR_SENCHK  InitialValue=false  ShowAdditionalParam=off  OutDataTypeStr=BOOL  Dimensions=1
  StartHold_Data : DataStoreMemory  Tag=POUVariable  Priority=10  DataStoreName=xxx_PLC_VAR_StartHold  InitialValue=false  ShowAdditionalParam=off  OutDataTypeStr=BOOL  Dimensions=1
  T_Data : DataStoreMemory  Tag=POUVariable  Priority=10  DataStoreName=xxx_PLC_VAR_T  InitialValue=TON_InitialValue  ShowAdditionalParam=off  OutDataTypeStr=Bus: TIMER  Dimensions=1
  TempS1HDown_Data : DataStoreMemory  Tag=POUVariable  Priority=10  DataStoreName=xxx_PLC_VAR_TempS1HDown  InitialValue=false  ShowAdditionalParam=off  OutDataTypeStr=BOOL  Dimensions=1
  TempS1HUp_Data : DataStoreMemory  Tag=POUVariable  Priority=10  DataStoreName=xxx_PLC_VAR_TempS1HUp  InitialValue=false  ShowAdditionalParam=off  OutDataTypeStr=BOOL  Dimensions=1
  TempS1H_Data : DataStoreMemory  Tag=POUVariable  Priority=10  DataStoreName=xxx_PLC_VAR_TempS1H  InitialValue=false  ShowAdditionalParam=off  OutDataTypeStr=BOOL  Dimensions=1
  TempS1Hup_Data : DataStoreMemory  Tag=POUVariable  Priority=10  DataStoreName=xxx_PLC_VAR_TempS1Hup  InitialValue=false  ShowAdditionalParam=off  OutDataTypeStr=BOOL  Dimensions=1
  TempS2HDown_Data : DataStoreMemory  Tag=POUVariable  Priority=10  DataStoreName=xxx_PLC_VAR_TempS2HDown  InitialValue=false  ShowAdditionalParam=off  OutDataTypeStr=BOOL  Dimensions=1
  TempS2HUp_Data : DataStoreMemory  Tag=POUVariable  Priority=10  DataStoreName=xxx_PLC_VAR_TempS2HUp  InitialValue=false  ShowAdditionalParam=off  OutDataTypeStr=BOOL  Dimensions=1
  TempS2H_Data : DataStoreMemory  Tag=POUVariable  Priority=10  DataStoreName=xxx_PLC_VAR_TempS2H  InitialValue=false  ShowAdditionalParam=off  OutDataTypeStr=BOOL  Dimensions=1
  TempS2LDown_Data : DataStoreMemory  Tag=POUVariable  Priority=10  DataStoreName=xxx_PLC_VAR_TempS2LDown  InitialValue=false  ShowAdditionalParam=off  OutDataTypeStr=BOOL  Dimensions=1
  TempS2LUp_Data : DataStoreMemory  Tag=POUVariable  Priority=10  DataStoreName=xxx_PLC_VAR_TempS2LUp  InitialValue=false  ShowAdditionalParam=off  OutDataTypeStr=BOOL  Dimensions=1
  TempS2L_Data : DataStoreMemory  Tag=POUVariable  Priority=10  DataStoreName=xxx_PLC_VAR_TempS2L  InitialValue=false  ShowAdditionalParam=off  OutDataTypeStr=BOOL  Dimensions=1
  TempS3LDown_Data : DataStoreMemory  Tag=POUVariable  Priority=10  DataStoreName=xxx_PLC_VAR_TempS3LDown  InitialValue=false  ShowAdditionalParam=off  OutDataTypeStr=BOOL  Dimensions=1
  TempS3LUp_Data : DataStoreMemory  Tag=POUVariable  Priority=10  DataStoreName=xxx_PLC_VAR_TempS3LUp  InitialValue=false  ShowAdditionalParam=off  OutDataTypeStr=BOOL  Dimensions=1
  TempS3L_Data : DataStoreMemory  Tag=POUVariable  Priority=10  DataStoreName=xxx_PLC_VAR_TempS3L  InitialValue=false  ShowAdditionalParam=off  OutDataTypeStr=BOOL  Dimensions=1
  VARVEL_Data : DataStoreMemory  Tag=POUVariable  Priority=10  DataStoreName=xxx_PLC_VAR_VARVEL  InitialValue=0.0  ShowAdditionalParam=off  OutDataTypeStr=single  Dimensions=1
  __Logic : Subsystem  Priority=12  TreatAsAtomicUnit=on
  _s4_3653__Block_Enable_Label : DataStoreMemory  Priority=10  DataStoreName=x_PLCLabel__s4_3653__Block_Enable  InitialValue=1  ShowAdditionalParam=off  OutDataTypeStr=BOOL  Dimensions=1
  _s4_3653__Block_Enable_LabelInitValue : Constant  OutDataTypeStr=BOOL
  _s4_3653__Block_Enable_LabelReset : DataStoreWrite  Priority=11  DataStoreName=x_PLCLabel__s4_3653__Block_Enable
  _s4_3653__Force_RungIn_False_Label : DataStoreMemory  Priority=10  DataStoreName=x_PLCLabel__s4_3653__Force_RungIn_False  ShowAdditionalParam=off  OutDataTypeStr=BOOL  Dimensions=1
  _s4_3653__Force_RungIn_False_LabelInitValue : Constant  Value=0  OutDataTypeStr=BOOL
  _s4_3653__Force_RungIn_False_LabelReset : DataStoreWrite  Priority=11  DataStoreName=x_PLCLabel__s4_3653__Force_RungIn_False
  _s4_3653__Variable_Write_Enable_Label : DataStoreMemory  Priority=10  DataStoreName=x_PLCLabel__s4_3653__Variable_Write_Enable  ShowAdditionalParam=off  OutDataTypeStr=BOOL  Dimensions=1
  _s4_3653__Variable_Write_Enable_LabelInitValue : Constant  Value=0  OutDataTypeStr=BOOL
  _s4_3653__Variable_Write_Enable_LabelReset : DataStoreWrite  Priority=11  DataStoreName=x_PLCLabel__s4_3653__Variable_Write_Enable
  wires:
  _s4_3653__Block_Enable_LabelInitValue/1 -> _s4_3653__Block_Enable_LabelReset/1
  _s4_3653__Variable_Write_Enable_LabelInitValue/1 -> _s4_3653__Variable_Write_Enable_LabelReset/1
  _s4_3653__Force_RungIn_False_LabelInitValue/1 -> _s4_3653__Force_RungIn_False_LabelReset/1

== system elevator/PLCControllerSuite/__Logic/Task/Up to Parent POU ==
